simulink library "halin"  (R2021b)
settings: Solver=VariableStepAuto  StartTime=0.0  StopTime=10.0  RelTol=1e-3
undefined symbols (not defined in the file): KHAL_CAN1ABM1E2E_flg, KHAL_CAN1EPB1E2E_flg, KHAL_CAN1EPS1E2E_flg, KHAL_CAN1ESC1E2E_flg, KHAL_CAN1ESC5E2E_flg, KHAL_CAN3BMS1E2E_flg, KHAL_CAN3BMS6E2E_flg, KHAL_CAN3CCU1E2E_flg, KHAL_CAN3CCU2E2E_flg, KHAL_CAN3MCUNF1E2E_flg, KHAL_CAN3MCUNR1E2E_flg, KHAL_CAN3Shifter1E2E_flg, KHAL_CAN3Shifter2E2E_flg, KHAL_CAN6FCM2E2E_flg, KHAL_CAN6FCM4E2E_flg, TRUE
libraries: simulink x645, FVT_lib x207, hcu_lib x59
(part 19 of 23)

== system halin/HAL_IN/CAN2/IVI2/IVIPSEATHeaterCmd ==
  IVI_PSEATHeater_Cmd : Inport
  UnitConverter : DataTypeConversion  OutDataTypeStr=uint8
  VHAL_IVIPSEATHeaterCmd_enum : Outport
  wires:
  UnitConverter/1 -> VHAL_IVIPSEATHeaterCmd_enum/1
  IVI_PSEATHeater_Cmd/1 -> UnitConverter/1

== system halin/HAL_IN/CAN2/IVI2/IVIPSEATReclineCmd ==
  IVI_PSEAT_Recline_Cmd : Inport
  UnitConverter : DataTypeConversion  OutDataTypeStr=uint8
  VHAL_IVIPSEATReclineCmd_enum : Outport
  wires:
  UnitConverter/1 -> VHAL_IVIPSEATReclineCmd_enum/1
  IVI_PSEAT_Recline_Cmd/1 -> UnitConverter/1

== system halin/HAL_IN/CAN2/IVI2/IVIPSEATSlideCmd ==
  IVI_PSEAT_Slide_Cmd : Inport
  UnitConverter : DataTypeConversion  OutDataTypeStr=uint8
  VHAL_IVIPSEATSlideCmd_enum : Outport
  wires:
  UnitConverter/1 -> VHAL_IVIPSEATSlideCmd_enum/1
  IVI_PSEAT_Slide_Cmd/1 -> UnitConverter/1

== system halin/HAL_IN/CAN2/IVI2/IVIPTGModeSW ==
  IVI_PTG_Mode_SW : Inport
  UnitConverter : DataTypeConversion  OutDataTypeStr=uint8
  VHAL_IVIPTGModeSW_enum : Outport
  wires:
  UnitConverter/1 -> VHAL_IVIPTGModeSW_enum/1
  IVI_PTG_Mode_SW/1 -> UnitConverter/1

== system halin/HAL_IN/CAN2/IVI2/IVIPTGOpenHeight ==
  IVI_PTG_Open_Height : Inport
  UnitConverter : DataTypeConversion  OutDataTypeStr=uint8
  VHAL_IVIPTGOpenHeight_enum : Outport
  wires:
  UnitConverter/1 -> VHAL_IVIPTGOpenHeight_enum/1
  IVI_PTG_Open_Height/1 -> UnitConverter/1

== system halin/HAL_IN/CAN2/IVI2/IVIPTGStaSW ==
  IVI_PTG_Sta_SW : Inport
  UnitConverter : DataTypeConversion  OutDataTypeStr=uint8
  VHAL_IVIPTGStaSW_enum : Outport
  wires:
  UnitConverter/1 -> VHAL_IVIPTGStaSW_enum/1
  IVI_PTG_Sta_SW/1 -> UnitConverter/1

== system halin/HAL_IN/CAN2/IVI2/IVIPTGUSStaSW ==
  IVI_PTG_USSta_SW : Inport
  UnitConverter : DataTypeConversion  OutDataTypeStr=uint8
  VHAL_IVIPTGUSStaSW_flg : Outport
  wires:
  UnitConverter/1 -> VHAL_IVIPTGUSStaSW_flg/1
  IVI_PTG_USSta_SW/1 -> UnitConverter/1

== system halin/HAL_IN/CAN2/IVI2/IVIPWModeReq ==
  IVI_PW_Mode_Req : Inport
  UnitConverter : DataTypeConversion  OutDataTypeStr=uint8
  VHAL_IVIPWModeReq_enum : Outport
  wires:
  UnitConverter/1 -> VHAL_IVIPWModeReq_enum/1
  IVI_PW_Mode_Req/1 -> UnitConverter/1

== system halin/HAL_IN/CAN2/IVI2/IVIPwrLockSW ==
  IVI_PwrLockSW : Inport
  UnitConverter : DataTypeConversion  OutDataTypeStr=uint8
  VHAL_IVIPwrLockSW_enum : Outport
  wires:
  UnitConverter/1 -> VHAL_IVIPwrLockSW_enum/1
  IVI_PwrLockSW/1 -> UnitConverter/1

== system halin/HAL_IN/CAN2/IVI2/IVIPwroffreq ==
  IVI_Pwroff_req : Inport
  UnitConverter : DataTypeConversion  OutDataTypeStr=uint8
  VHAL_IVIPwroffreq_flg : Outport
  wires:
  UnitConverter/1 -> VHAL_IVIPwroffreq_flg/1
  IVI_Pwroff_req/1 -> UnitConverter/1

== system halin/HAL_IN/CAN2/IVI2/IVIRRDefReq ==
  IVI_RR_Def_Req : Inport
  UnitConverter : DataTypeConversion  OutDataTypeStr=uint8
  VHAL_IVIRRDefReq_flg : Outport
  wires:
  UnitConverter/1 -> VHAL_IVIRRDefReq_flg/1
  IVI_RR_Def_Req/1 -> UnitConverter/1

== system halin/HAL_IN/CAN2/IVI2/IVIReqV2L ==
  IVI_Req_V2L : Inport
  UnitConverter : DataTypeConversion  OutDataTypeStr=uint8
  VHAL_IVIReqV2L_enum : Outport
  wires:
  UnitConverter/1 -> VHAL_IVIReqV2L_enum/1
  IVI_Req_V2L/1 -> UnitConverter/1

== system halin/HAL_IN/CAN2/IVI2/IVISWCRUndefinedSta ==
  IVI_SWC_RUndefined_Sta : Inport
  UnitConverter : DataTypeConversion  OutDataTypeStr=uint8
  VHAL_IVISWCRUndefinedSta_enum : Outport
  wires:
  UnitConverter/1 -> VHAL_IVISWCRUndefinedSta_enum/1
  IVI_SWC_RUndefined_Sta/1 -> UnitConverter/1

== system halin/HAL_IN/CAN2/IVI2/IVIScreen ==
  IVI_Screen : Inport
  UnitConverter : DataTypeConversion  OutDataTypeStr=uint8
  VHAL_IVIScreen_enum : Outport
  wires:
  UnitConverter/1 -> VHAL_IVIScreen_enum/1
  IVI_Screen/1 -> UnitConverter/1

== system halin/HAL_IN/CAN2/IVI2/IVIStartChgreq ==
  IVI_Start_Chg_req : Inport
  UnitConverter : DataTypeConversion  OutDataTypeStr=uint8
  VHAL_IVIStartChgreq_flg : Outport
  wires:
  UnitConverter/1 -> VHAL_IVIStartChgreq_flg/1
  IVI_Start_Chg_req/1 -> UnitConverter/1

== system halin/HAL_IN/CAN2/IVI2/IVIStatus ==
  IVI_Status : Inport
  UnitConverter : DataTypeConversion  OutDataTypeStr=uint8
  VHAL_IVIStatus_flg : Outport
  wires:
  UnitConverter/1 -> VHAL_IVIStatus_flg/1
  IVI_Status/1 -> UnitConverter/1

== system halin/HAL_IN/CAN2/IVI2/IVIStopChgreq ==
  IVI_Stop_Chg_req : Inport
  UnitConverter : DataTypeConversion  OutDataTypeStr=uint8
  VHAL_IVIStopChgreq_flg : Outport
  wires:
  UnitConverter/1 -> VHAL_IVIStopChgreq_flg/1
  IVI_Stop_Chg_req/1 -> UnitConverter/1

== system halin/HAL_IN/CAN2/IVI2/IVITrailerCheckReqSta ==
  IVI_TrailerCheckReq_Sta : Inport
  UnitConverter : DataTypeConversion  OutDataTypeStr=uint8
  VHAL_IVITrailerCheckReqSta_flg : Outport
  wires:
  UnitConverter/1 -> VHAL_IVITrailerCheckReqSta_flg/1
  IVI_TrailerCheckReq_Sta/1 -> UnitConverter/1

== system halin/HAL_IN/CAN2/IVI2/IVITrailerModeSWSta ==
  IVI_TrailerModeSW_Sta : Inport
  UnitConverter : DataTypeConversion  OutDataTypeStr=uint8
  VHAL_IVITrailerModeSWSta_flg : Outport
  wires:
  UnitConverter/1 -> VHAL_IVITrailerModeSWSta_flg/1
  IVI_TrailerModeSW_Sta/1 -> UnitConverter/1

== system halin/HAL_IN/CAN2/IVI2/IVITriggerreq ==
  IVI_Trigger_req : Inport
  UnitConverter : DataTypeConversion  OutDataTypeStr=uint8
  VHAL_IVITriggerreq_flg : Outport
  wires:
  UnitConverter/1 -> VHAL_IVITriggerreq_flg/1
  IVI_Trigger_req/1 -> UnitConverter/1

== system halin/HAL_IN/CAN2/IVI2/IVIUnlockChgreq ==
  IVI_Unlock_Chg_req : Inport
  UnitConverter : DataTypeConversion  OutDataTypeStr=uint8
  VHAL_IVIUnlockChgreq_flg : Outport
  wires:
  UnitConverter/1 -> VHAL_IVIUnlockChgreq_flg/1
  IVI_Unlock_Chg_req/1 -> UnitConverter/1

== system halin/HAL_IN/CAN2/IVI2/IVIWIMAINSW ==
  IVI_WI_MAIN_SW : Inport
  UnitConverter : DataTypeConversion  OutDataTypeStr=uint8
  VHAL_IVIWIMAINSW_flg : Outport
  wires:
  UnitConverter/1 -> VHAL_IVIWIMAINSW_flg/1
  IVI_WI_MAIN_SW/1 -> UnitConverter/1

== system halin/HAL_IN/CAN2/IVI2/LDrvControlCommand ==
  L_Drv_ControlCommand : Inport
  UnitConverter : DataTypeConversion  OutDataTypeStr=uint8
  VHAL_LDrvControlCommand_pct : Outport
  wires:
  UnitConverter/1 -> VHAL_LDrvControlCommand_pct/1
  L_Drv_ControlCommand/1 -> UnitConverter/1

== system halin/HAL_IN/CAN2/IVI2/LPasControlCommand ==
  L_Pas_ControlCommand : Inport
  UnitConverter : DataTypeConversion  OutDataTypeStr=uint8
  VHAL_LPasControlCommand_pct : Outport
  wires:
  UnitConverter/1 -> VHAL_LPasControlCommand_pct/1
  L_Pas_ControlCommand/1 -> UnitConverter/1

== system halin/HAL_IN/CAN2/IVI2/LRLDControlCommand ==
  L_RLD_ControlCommand : Inport
  UnitConverter : DataTypeConversion  OutDataTypeStr=uint8
  VHAL_LRLDControlCommand_pct : Outport
  wires:
  UnitConverter/1 -> VHAL_LRLDControlCommand_pct/1
  L_RLD_ControlCommand/1 -> UnitConverter/1

== system halin/HAL_IN/CAN2/IVI2/LRRDControlCommand ==
  L_RRD_ControlCommand : Inport
  UnitConverter : DataTypeConversion  OutDataTypeStr=uint8
  VHAL_LRRDControlCommand_pct : Outport
  wires:
  UnitConverter/1 -> VHAL_LRRDControlCommand_pct/1
  L_RRD_ControlCommand/1 -> UnitConverter/1

== system halin/HAL_IN/CAN2/IVI2/LightShowStartReq ==
  Light_ShowStart_Req : Inport
  UnitConverter : DataTypeConversion  OutDataTypeStr=uint8
  VHAL_LightShowStartReq_flg : Outport
  wires:
  UnitConverter/1 -> VHAL_LightShowStartReq_flg/1
  Light_ShowStart_Req/1 -> UnitConverter/1

== system halin/HAL_IN/CAN2/IVI2/LightShowStopReq ==
  Light_ShowStop_Req : Inport
  UnitConverter : DataTypeConversion  OutDataTypeStr=uint8
  VHAL_LightShowStopReq_flg : Outport
  wires:
  UnitConverter/1 -> VHAL_LightShowStopReq_flg/1
  Light_ShowStop_Req/1 -> UnitConverter/1

== system halin/HAL_IN/CAN2/IVI2/MFRDNBrightReq ==
  MFRD_N_Bright_Req : Inport
  UnitConverter : DataTypeConversion  OutDataTypeStr=uint8
  VHAL_MFRDNBrightReq_pct : Outport
  wires:
  UnitConverter/1 -> VHAL_MFRDNBrightReq_pct/1
  MFRD_N_Bright_Req/1 -> UnitConverter/1

== system halin/HAL_IN/CAN2/IVI2/OFFACMODE ==
  OFF_AC_MODE : Inport
  UnitConverter : DataTypeConversion  OutDataTypeStr=uint8
  VHAL_OFFACMODE_enum : Outport
  wires:
  UnitConverter/1 -> VHAL_OFFACMODE_enum/1
  OFF_AC_MODE/1 -> UnitConverter/1

== system halin/HAL_IN/CAN2/IVI2/PSEATventreq ==
  PSEAT_vent_req : Inport
  UnitConverter : DataTypeConversion  OutDataTypeStr=uint8
  VHAL_PSEATventreq_enum : Outport
  wires:
  UnitConverter/1 -> VHAL_PSEATventreq_enum/1
  PSEAT_vent_req/1 -> UnitConverter/1

== system halin/HAL_IN/CAN2/IVI2/PerdV2L ==
  Perd_V2L : Inport
  UnitConverter : DataTypeConversion  OutDataTypeStr=uint8
  VHAL_PerdV2L_enum : Outport
  wires:
  UnitConverter/1 -> VHAL_PerdV2L_enum/1
  Perd_V2L/1 -> UnitConverter/1

== system halin/HAL_IN/CAN2/IVI2/RFogLampSW ==
  RFogLampSW : Inport
  UnitConverter : DataTypeConversion  OutDataTypeStr=uint8
  VHAL_RFogLampSW_flg : Outport
  wires:
  UnitConverter/1 -> VHAL_RFogLampSW_flg/1
  RFogLampSW/1 -> UnitConverter/1

== system halin/HAL_IN/CAN2/IVI2/RollModeSWCmd ==
  Roll_Mode_SW_Cmd : Inport
  UnitConverter : DataTypeConversion  OutDataTypeStr=uint8
  VHAL_RollModeSWCmd_enum : Outport
  wires:
  UnitConverter/1 -> VHAL_RollModeSWCmd_enum/1
  Roll_Mode_SW_Cmd/1 -> UnitConverter/1

== system halin/HAL_IN/CAN2/IVI2/RoomLampMode ==
  RoomLampMode : Inport
  UnitConverter : DataTypeConversion  OutDataTypeStr=uint8
  VHAL_RoomLampMode_flg : Outport
  wires:
  UnitConverter/1 -> VHAL_RoomLampMode_flg/1
  RoomLampMode/1 -> UnitConverter/1

== system halin/HAL_IN/CAN2/IVI2/SOCADJBUTT ==
  SOC_ADJ_BUTT : Inport
  UnitConverter : DataTypeConversion  OutDataTypeStr=uint8
  VHAL_SOCADJBUTT_flg : Outport
  wires:
  UnitConverter/1 -> VHAL_SOCADJBUTT_flg/1
  SOC_ADJ_BUTT/1 -> UnitConverter/1

== system halin/HAL_IN/CAN2/IVI2/SOCLimitSet ==
  SOC_Limit_Set : Inport
  UnitConverter : DataTypeConversion  OutDataTypeStr=uint8
  convert_in : FVT_lib/hal/convert_in  gain=2  offset=50
  VHAL_SOCLimitSet_pct : Outport
  wires:
  convert_in/1 -> VHAL_SOCLimitSet_pct/1
  UnitConverter/1 -> convert_in/1
  SOC_Limit_Set/1 -> UnitConverter/1

== system halin/HAL_IN/CAN2/IVI2/SOCV2LLimit ==
  SOC_V2LLimit : Inport
  UnitConverter : DataTypeConversion  OutDataTypeStr=uint8
  VHAL_SOCV2LLimit_pct : Outport
  wires:
  UnitConverter/1 -> VHAL_SOCV2LLimit_pct/1
  SOC_V2LLimit/1 -> UnitConverter/1

== system halin/HAL_IN/CAN2/IVI2/SchedChgStart ==
  Sched_Chg_Start : Inport
  UnitConverter : DataTypeConversion  OutDataTypeStr=uint8
  VHAL_SchedChgStart_flg : Outport
  wires:
  UnitConverter/1 -> VHAL_SchedChgStart_flg/1
  Sched_Chg_Start/1 -> UnitConverter/1

== system halin/HAL_IN/CAN2/IVI2/SchedChgStop ==
  Sched_Chg_Stop : Inport
  UnitConverter : DataTypeConversion  OutDataTypeStr=uint8
  VHAL_SchedChgStop_flg : Outport
  wires:
  UnitConverter/1 -> VHAL_SchedChgStop_flg/1
  Sched_Chg_Stop/1 -> UnitConverter/1

== system halin/HAL_IN/CAN2/IVI2/SchedChgbutt ==
  Sched_Chg_butt : Inport
  UnitConverter : DataTypeConversion  OutDataTypeStr=uint8
  VHAL_SchedChgbutt_flg : Outport
  wires:
  UnitConverter/1 -> VHAL_SchedChgbutt_flg/1
  Sched_Chg_butt/1 -> UnitConverter/1

== system halin/HAL_IN/CAN2/IVI2/SchedChglimit ==
  Sched_Chg_limit : Inport
  UnitConverter : DataTypeConversion  OutDataTypeStr=uint8
  convert_in : FVT_lib/hal/convert_in  gain=2  offset=50
  VHAL_SchedChglimit_pct : Outport
  wires:
  convert_in/1 -> VHAL_SchedChglimit_pct/1
  UnitConverter/1 -> convert_in/1
  Sched_Chg_limit/1 -> UnitConverter/1

== system halin/HAL_IN/CAN2/IVI2/SchedChgwake ==
  Sched_Chg_wake : Inport
  UnitConverter : DataTypeConversion  OutDataTypeStr=uint8
  VHAL_SchedChgwake_flg : Outport
  wires:
  UnitConverter/1 -> VHAL_SchedChgwake_flg/1
  Sched_Chg_wake/1 -> UnitConverter/1

== system halin/HAL_IN/CAN2/IVI2/SenstivityPosition ==
  SenstivityPosition : Inport
  UnitConverter : DataTypeConversion  OutDataTypeStr=uint8
  VHAL_SenstivityPosition_enum : Outport
  wires:
  UnitConverter/1 -> VHAL_SenstivityPosition_enum/1
  SenstivityPosition/1 -> UnitConverter/1

== system halin/HAL_IN/CAN2/IVI2/SetUnlockSingle ==
  SetUnlockSingle : Inport
  UnitConverter : DataTypeConversion  OutDataTypeStr=uint8
  VHAL_SetUnlockSingle_flg : Outport
  wires:
  UnitConverter/1 -> VHAL_SetUnlockSingle_flg/1
  SetUnlockSingle/1 -> UnitConverter/1

== system halin/HAL_IN/CAN2/IVI2/TCSSWCmd ==
  TCS_SW_Cmd : Inport
  UnitConverter : DataTypeConversion  OutDataTypeStr=uint8
  VHAL_TCSSWCmd_enum : Outport
  wires:
  UnitConverter/1 -> VHAL_TCSSWCmd_enum/1
  TCS_SW_Cmd/1 -> UnitConverter/1

== system halin/HAL_IN/CAN2/IVI2/TPMSCaliButt ==
  TPMS_Cali_Butt : Inport
  UnitConverter : DataTypeConversion  OutDataTypeStr=uint8
  VHAL_TPMSCaliButt_flg : Outport
  wires:
  UnitConverter/1 -> VHAL_TPMSCaliButt_flg/1
  TPMS_Cali_Butt/1 -> UnitConverter/1

== system halin/HAL_IN/CAN2/IVI2/TPMSResButt ==
  TPMS_Res_Butt : Inport
  UnitConverter : DataTypeConversion  OutDataTypeStr=uint8
  VHAL_TPMSResButt_flg : Outport
  wires:
  UnitConverter/1 -> VHAL_TPMSResButt_flg/1
  TPMS_Res_Butt/1 -> UnitConverter/1

== system halin/HAL_IN/CAN2/IVI2/TurnSwTimeSet ==
  TurnSwTimeSet : Inport
  UnitConverter : DataTypeConversion  OutDataTypeStr=uint8
  VHAL_TurnSwTimeSet_enum : Outport
  wires:
  UnitConverter/1 -> VHAL_TurnSwTimeSet_enum/1
  TurnSwTimeSet/1 -> UnitConverter/1

== system halin/HAL_IN/CAN2/IVI2/WalkawayLockSW ==
  Walkaway_Lock_SW : Inport
  UnitConverter : DataTypeConversion  OutDataTypeStr=uint8
  VHAL_WalkawayLockSW_flg : Outport
  wires:
  UnitConverter/1 -> VHAL_WalkawayLockSW_flg/1
  Walkaway_Lock_SW/1 -> UnitConverter/1

== system halin/HAL_IN/CAN2/IVI2/WlcmLightMode ==
  WlcmLight_Mode : Inport
  UnitConverter : DataTypeConversion  OutDataTypeStr=uint8
  VHAL_WlcmLightMode_enum : Outport
  wires:
  UnitConverter/1 -> VHAL_WlcmLightMode_enum/1
  WlcmLight_Mode/1 -> UnitConverter/1

== system halin/HAL_IN/CAN2/IVI2/sigAirIntenZon1Req ==
  sigAirIntenZon1Req : Inport
  UnitConverter : DataTypeConversion  OutDataTypeStr=uint8
  VHAL_sigAirIntenZon1Req_enum : Outport
  wires:
  UnitConverter/1 -> VHAL_sigAirIntenZon1Req_enum/1
  sigAirIntenZon1Req/1 -> UnitConverter/1

== system halin/HAL_IN/CAN2/IVI2/sigDfrstReq ==
  sigDfrstReq : Inport
  UnitConverter : DataTypeConversion  OutDataTypeStr=uint8
  VHAL_sigDfrstReq_flg : Outport
  wires:
  UnitConverter/1 -> VHAL_sigDfrstReq_flg/1
  sigDfrstReq/1 -> UnitConverter/1

== system halin/HAL_IN/CAN2/IVI2/sigFaceReq ==
  sigFaceReq : Inport
  UnitConverter : DataTypeConversion  OutDataTypeStr=uint8
  VHAL_sigFaceReq_flg : Outport
  wires:
  UnitConverter/1 -> VHAL_sigFaceReq_flg/1
  sigFaceReq/1 -> UnitConverter/1

== system halin/HAL_IN/CAN2/IVI2/sigFootReq ==
  sigFootReq : Inport
  UnitConverter : DataTypeConversion  OutDataTypeStr=uint8
  VHAL_sigFootReq_flg : Outport
  wires:
  UnitConverter/1 -> VHAL_sigFootReq_flg/1
  sigFootReq/1 -> UnitConverter/1

== system halin/HAL_IN/CAN2/IVI2/sigRecircReq ==
  sigRecircReq : Inport
  UnitConverter : DataTypeConversion  OutDataTypeStr=uint8
  VHAL_sigRecircReq_flg : Outport
  wires:
  UnitConverter/1 -> VHAL_sigRecircReq_flg/1
  sigRecircReq/1 -> UnitConverter/1

== system halin/HAL_IN/CAN2/IVI2/sigSetTempZon1Req ==
  sigSetTempZon1Req : Inport
  UnitConverter : DataTypeConversion  OutDataTypeStr=uint8
  convert_in : FVT_lib/hal/convert_in  gain=0.5  offset=17
  VHAL_sigSetTempZon1Req_C : Outport
  wires:
  convert_in/1 -> VHAL_sigSetTempZon1Req_C/1
  UnitConverter/1 -> convert_in/1
  sigSetTempZon1Req/1 -> UnitConverter/1

== system halin/HAL_IN/CAN2/IVI2/sigSetTempZon2Req ==
  sigSetTempZon2Req : Inport
  UnitConverter : DataTypeConversion  OutDataTypeStr=uint8
  convert_in : FVT_lib/hal/convert_in  gain=0.5  offset=17
  VHAL_sigSetTempZon2Req_C : Outport
  wires:
  convert_in/1 -> VHAL_sigSetTempZon2Req_C/1
  UnitConverter/1 -> convert_in/1
  sigSetTempZon2Req/1 -> UnitConverter/1

== system halin/HAL_IN/CAN2/IVI3/IVICLBlowerYSta ==
  IVI_CLBlower_Y_Sta : Inport
  UnitConverter : DataTypeConversion  OutDataTypeStr=uint8
  VHAL_IVICLBlowerYSta_pct : Outport
  wires:
  UnitConverter/1 -> VHAL_IVICLBlowerYSta_pct/1
  IVI_CLBlower_Y_Sta/1 -> UnitConverter/1

== system halin/HAL_IN/CAN2/IVI3/IVICLBlowerZSta ==
  IVI_CLBlower_Z_Sta : Inport
  UnitConverter : DataTypeConversion  OutDataTypeStr=uint8
  VHAL_IVICLBlowerZSta_pct : Outport
  wires:
  UnitConverter/1 -> VHAL_IVICLBlowerZSta_pct/1
  IVI_CLBlower_Z_Sta/1 -> UnitConverter/1

== system halin/HAL_IN/CAN2/IVI3/IVICRBlowerYSta ==
  IVI_CRBlower_Y_Sta : Inport
  UnitConverter : DataTypeConversion  OutDataTypeStr=uint8
  VHAL_IVICRBlowerYSta_pct : Outport
  wires:
  UnitConverter/1 -> VHAL_IVICRBlowerYSta_pct/1
  IVI_CRBlower_Y_Sta/1 -> UnitConverter/1

== system halin/HAL_IN/CAN2/IVI3/IVICRBlowerZSta ==
  IVI_CRBlower_Z_Sta : Inport
  UnitConverter : DataTypeConversion  OutDataTypeStr=uint8
  VHAL_IVICRBlowerZSta_pct : Outport
  wires:
  UnitConverter/1 -> VHAL_IVICRBlowerZSta_pct/1
  IVI_CRBlower_Z_Sta/1 -> UnitConverter/1

== system halin/HAL_IN/CAN2/IVI3/IVIDrBlowerModeSta ==
  IVI_DrBlower_Mode_Sta : Inport
  UnitConverter : DataTypeConversion  OutDataTypeStr=uint8
  VHAL_IVIDrBlowerModeSta_enum : Outport
  wires:
  UnitConverter/1 -> VHAL_IVIDrBlowerModeSta_enum/1
  IVI_DrBlower_Mode_Sta/1 -> UnitConverter/1

== system halin/HAL_IN/CAN2/IVI3/IVIDrBlowerYSta ==
  IVI_DrBlower_Y_Sta : Inport
  UnitConverter : DataTypeConversion  OutDataTypeStr=uint8
  VHAL_IVIDrBlowerYSta_pct : Outport
  wires:
  UnitConverter/1 -> VHAL_IVIDrBlowerYSta_pct/1
  IVI_DrBlower_Y_Sta/1 -> UnitConverter/1

== system halin/HAL_IN/CAN2/IVI3/IVIDrBlowerZSta ==
  IVI_DrBlower_Z_Sta : Inport
  UnitConverter : DataTypeConversion  OutDataTypeStr=uint8
  VHAL_IVIDrBlowerZSta_pct : Outport
  wires:
  UnitConverter/1 -> VHAL_IVIDrBlowerZSta_pct/1
  IVI_DrBlower_Z_Sta/1 -> UnitConverter/1

== system halin/HAL_IN/CAN2/IVI3/IVIHMICustmiFunSta ==
  IVI_HMI_CustmiFun_Sta : Inport
  UnitConverter : DataTypeConversion  OutDataTypeStr=uint8
  VHAL_IVIHMICustmiFunSta_enum : Outport
  wires:
  UnitConverter/1 -> VHAL_IVIHMICustmiFunSta_enum/1
  IVI_HMI_CustmiFun_Sta/1 -> UnitConverter/1

== system halin/HAL_IN/CAN2/IVI3/IVIHMICustmiKEYSta ==
  IVI_HMI_CustmiKEY_Sta : Inport
  UnitConverter : DataTypeConversion  OutDataTypeStr=uint8
  VHAL_IVIHMICustmiKEYSta_enum : Outport
  wires:
  UnitConverter/1 -> VHAL_IVIHMICustmiKEYSta_enum/1
  IVI_HMI_CustmiKEY_Sta/1 -> UnitConverter/1

== system halin/HAL_IN/CAN2/IVI3/IVILSEATventCmd ==
  IVI_LSEATvent_Cmd : Inport
  UnitConverter : DataTypeConversion  OutDataTypeStr=uint8
  VHAL_IVILSEATventCmd_enum : Outport
  wires:
  UnitConverter/1 -> VHAL_IVILSEATventCmd_enum/1
  IVI_LSEATvent_Cmd/1 -> UnitConverter/1

== system halin/HAL_IN/CAN2/IVI3/IVIMLFMostCmd ==
  IVI_MLFMost_Cmd : Inport
  UnitConverter : DataTypeConversion  OutDataTypeStr=uint8
  VHAL_IVIMLFMostCmd_flg : Outport
  wires:
  UnitConverter/1 -> VHAL_IVIMLFMostCmd_flg/1
  IVI_MLFMost_Cmd/1 -> UnitConverter/1

== system halin/HAL_IN/CAN2/IVI3/IVIMLFootLiftCmd ==
  IVI_MLFootLift_Cmd : Inport
  UnitConverter : DataTypeConversion  OutDataTypeStr=uint8
  VHAL_IVIMLFootLiftCmd_enum : Outport
  wires:
  UnitConverter/1 -> VHAL_IVIMLFootLiftCmd_enum/1
  IVI_MLFootLift_Cmd/1 -> UnitConverter/1

== system halin/HAL_IN/CAN2/IVI3/IVIMLNapModeCmd ==
  IVI_MLNapMode_Cmd : Inport
  UnitConverter : DataTypeConversion  OutDataTypeStr=uint8
  VHAL_IVIMLNapModeCmd_flg : Outport
  wires:
  UnitConverter/1 -> VHAL_IVIMLNapModeCmd_flg/1
  IVI_MLNapMode_Cmd/1 -> UnitConverter/1

== system halin/HAL_IN/CAN2/IVI3/IVIMLReclinerCmd ==
  IVI_MLRecliner_Cmd : Inport
  UnitConverter : DataTypeConversion  OutDataTypeStr=uint8
  VHAL_IVIMLReclinerCmd_enum : Outport
  wires:
  UnitConverter/1 -> VHAL_IVIMLReclinerCmd_enum/1
  IVI_MLRecliner_Cmd/1 -> UnitConverter/1

== system halin/HAL_IN/CAN2/IVI3/IVIMLRestoreCmd ==
  IVI_MLRestore_Cmd : Inport
  UnitConverter : DataTypeConversion  OutDataTypeStr=uint8
  VHAL_IVIMLRestoreCmd_flg : Outport
  wires:
  UnitConverter/1 -> VHAL_IVIMLRestoreCmd_flg/1
  IVI_MLRestore_Cmd/1 -> UnitConverter/1

== system halin/HAL_IN/CAN2/IVI3/IVIMLSEATventCmd ==
  IVI_MLSEATvent_Cmd : Inport
  UnitConverter : DataTypeConversion  OutDataTypeStr=uint8
  VHAL_IVIMLSEATventCmd_enum : Outport
  wires:
  UnitConverter/1 -> VHAL_IVIMLSEATventCmd_enum/1
  IVI_MLSEATvent_Cmd/1 -> UnitConverter/1

== system halin/HAL_IN/CAN2/IVI3/IVIMLSeatLiftCmd ==
  IVI_MLSeatLift_Cmd : Inport
  UnitConverter : DataTypeConversion  OutDataTypeStr=uint8
  VHAL_IVIMLSeatLiftCmd_enum : Outport
  wires:
  UnitConverter/1 -> VHAL_IVIMLSeatLiftCmd_enum/1
  IVI_MLSeatLift_Cmd/1 -> UnitConverter/1

== system halin/HAL_IN/CAN2/IVI3/IVIMLSldRestoreCmd ==
  IVI_MLSldRestore_Cmd : Inport
  UnitConverter : DataTypeConversion  OutDataTypeStr=uint8
  VHAL_IVIMLSldRestoreCmd_flg : Outport
  wires:
  UnitConverter/1 -> VHAL_IVIMLSldRestoreCmd_flg/1
  IVI_MLSldRestore_Cmd/1 -> UnitConverter/1

== system halin/HAL_IN/CAN2/IVI3/IVIMLSliderCmd ==
  IVI_MLSlider_Cmd : Inport
  UnitConverter : DataTypeConversion  OutDataTypeStr=uint8
  VHAL_IVIMLSliderCmd_enum : Outport
  wires:
  UnitConverter/1 -> VHAL_IVIMLSliderCmd_enum/1
  IVI_MLSlider_Cmd/1 -> UnitConverter/1

== system halin/HAL_IN/CAN2/IVI3/IVIMLZeroGravityCmd ==
  IVI_MLZeroGravity_Cmd : Inport
  UnitConverter : DataTypeConversion  OutDataTypeStr=uint8
  VHAL_IVIMLZeroGravityCmd_flg : Outport
  wires:
  UnitConverter/1 -> VHAL_IVIMLZeroGravityCmd_flg/1
  IVI_MLZeroGravity_Cmd/1 -> UnitConverter/1

== system halin/HAL_IN/CAN2/IVI3/IVIMRFMostCmd ==
  IVI_MRFMost_Cmd : Inport
  UnitConverter : DataTypeConversion  OutDataTypeStr=uint8
  VHAL_IVIMRFMostCmd_flg : Outport
  wires:
  UnitConverter/1 -> VHAL_IVIMRFMostCmd_flg/1
  IVI_MRFMost_Cmd/1 -> UnitConverter/1

== system halin/HAL_IN/CAN2/IVI3/IVIMRFootLiftCmd ==
  IVI_MRFootLift_Cmd : Inport
  UnitConverter : DataTypeConversion  OutDataTypeStr=uint8
  VHAL_IVIMRFootLiftCmd_enum : Outport
  wires:
  UnitConverter/1 -> VHAL_IVIMRFootLiftCmd_enum/1
  IVI_MRFootLift_Cmd/1 -> UnitConverter/1

== system halin/HAL_IN/CAN2/IVI3/IVIMRNapModeCmd ==
  IVI_MRNapMode_Cmd : Inport
  UnitConverter : DataTypeConversion  OutDataTypeStr=uint8
  VHAL_IVIMRNapModeCmd_flg : Outport
  wires:
  UnitConverter/1 -> VHAL_IVIMRNapModeCmd_flg/1
  IVI_MRNapMode_Cmd/1 -> UnitConverter/1

== system halin/HAL_IN/CAN2/IVI3/IVIMRReclinerCmd ==
  IVI_MRRecliner_Cmd : Inport
  UnitConverter : DataTypeConversion  OutDataTypeStr=uint8
  VHAL_IVIMRReclinerCmd_enum : Outport
  wires:
  UnitConverter/1 -> VHAL_IVIMRReclinerCmd_enum/1
  IVI_MRRecliner_Cmd/1 -> UnitConverter/1

== system halin/HAL_IN/CAN2/IVI3/IVIMRRestoreCmd ==
  IVI_MRRestore_Cmd : Inport
  UnitConverter : DataTypeConversion  OutDataTypeStr=uint8
  VHAL_IVIMRRestoreCmd_flg : Outport
  wires:
  UnitConverter/1 -> VHAL_IVIMRRestoreCmd_flg/1
  IVI_MRRestore_Cmd/1 -> UnitConverter/1

== system halin/HAL_IN/CAN2/IVI3/IVIMRSEATventCmd ==
  IVI_MRSEATvent_Cmd : Inport
  UnitConverter : DataTypeConversion  OutDataTypeStr=uint8
  VHAL_IVIMRSEATventCmd_enum : Outport
  wires:
  UnitConverter/1 -> VHAL_IVIMRSEATventCmd_enum/1
  IVI_MRSEATvent_Cmd/1 -> UnitConverter/1

== system halin/HAL_IN/CAN2/IVI3/IVIMRSeatLiftCmd ==
  IVI_MRSeatLift_Cmd : Inport
  UnitConverter : DataTypeConversion  OutDataTypeStr=uint8
  VHAL_IVIMRSeatLiftCmd_enum : Outport
  wires:
  UnitConverter/1 -> VHAL_IVIMRSeatLiftCmd_enum/1
  IVI_MRSeatLift_Cmd/1 -> UnitConverter/1

== system halin/HAL_IN/CAN2/IVI3/IVIMRSldRestoreCmd ==
  IVI_MRSldRestore_Cmd : Inport
  UnitConverter : DataTypeConversion  OutDataTypeStr=uint8
  VHAL_IVIMRSldRestoreCmd_flg : Outport
  wires:
  UnitConverter/1 -> VHAL_IVIMRSldRestoreCmd_flg/1
  IVI_MRSldRestore_Cmd/1 -> UnitConverter/1

== system halin/HAL_IN/CAN2/IVI3/IVIMRSliderCmd ==
  IVI_MRSlider_Cmd : Inport
  UnitConverter : DataTypeConversion  OutDataTypeStr=uint8
  VHAL_IVIMRSliderCmd_enum : Outport
  wires:
  UnitConverter/1 -> VHAL_IVIMRSliderCmd_enum/1
  IVI_MRSlider_Cmd/1 -> UnitConverter/1

== system halin/HAL_IN/CAN2/IVI3/IVIMRZeroGravityCmd ==
  IVI_MRZeroGravity_Cmd : Inport
  UnitConverter : DataTypeConversion  OutDataTypeStr=uint8
  VHAL_IVIMRZeroGravityCmd_flg : Outport
  wires:
  UnitConverter/1 -> VHAL_IVIMRZeroGravityCmd_flg/1
  IVI_MRZeroGravity_Cmd/1 -> UnitConverter/1

== system halin/HAL_IN/CAN2/IVI3/IVIPsBlowerModeSta ==
  IVI_PsBlower_Mode_Sta : Inport
  UnitConverter : DataTypeConversion  OutDataTypeStr=uint8
  VHAL_IVIPsBlowerModeSta_enum : Outport
  wires:
  UnitConverter/1 -> VHAL_IVIPsBlowerModeSta_enum/1
  IVI_PsBlower_Mode_Sta/1 -> UnitConverter/1

== system halin/HAL_IN/CAN2/IVI3/IVIPsBlowerYSta ==
  IVI_PsBlower_Y_Sta : Inport
  UnitConverter : DataTypeConversion  OutDataTypeStr=uint8
  VHAL_IVIPsBlowerYSta_pct : Outport
  wires:
  UnitConverter/1 -> VHAL_IVIPsBlowerYSta_pct/1
  IVI_PsBlower_Y_Sta/1 -> UnitConverter/1

== system halin/HAL_IN/CAN2/IVI3/IVIPsBlowerZSta ==
  IVI_PsBlower_Z_Sta : Inport
  UnitConverter : DataTypeConversion  OutDataTypeStr=uint8
  VHAL_IVIPsBlowerZSta_pct : Outport
  wires:
  UnitConverter/1 -> VHAL_IVIPsBlowerZSta_pct/1
  IVI_PsBlower_Z_Sta/1 -> UnitConverter/1

== system halin/HAL_IN/CAN2/IVI3/IVIRSEATventCmd ==
  IVI_RSEATvent_Cmd : Inport
  UnitConverter : DataTypeConversion  OutDataTypeStr=uint8
  VHAL_IVIRSEATventCmd_enum : Outport
  wires:
  UnitConverter/1 -> VHAL_IVIRSEATventCmd_enum/1
  IVI_RSEATvent_Cmd/1 -> UnitConverter/1

== system halin/HAL_IN/CAN2/IVI3/IVISnowModeCmd ==
  IVI_SnowMode_Cmd : Inport
  UnitConverter : DataTypeConversion  OutDataTypeStr=uint8
  VHAL_IVISnowModeCmd_flg : Outport
  wires:
  UnitConverter/1 -> VHAL_IVISnowModeCmd_flg/1
  IVI_SnowMode_Cmd/1 -> UnitConverter/1

== system halin/HAL_IN/CAN2/IVI3/IVIUserTakeOverAPSSta ==
  IVI_UserTakeOver_APS_Sta : Inport
  UnitConverter : DataTypeConversion  OutDataTypeStr=uint8
  VHAL_IVIUserTakeOverAPSSta_flg : Outport
  wires:
  UnitConverter/1 -> VHAL_IVIUserTakeOverAPSSta_flg/1
  IVI_UserTakeOver_APS_Sta/1 -> UnitConverter/1

== system halin/HAL_IN/CAN2/IVI3/IVIZon1WindDirSWReqSta ==
  IVI_Zon1WindDirSWReq_Sta : Inport
  UnitConverter : DataTypeConversion  OutDataTypeStr=uint8
  VHAL_IVIZon1WindDirSWReqSta_flg : Outport
  wires:
  UnitConverter/1 -> VHAL_IVIZon1WindDirSWReqSta_flg/1
  IVI_Zon1WindDirSWReq_Sta/1 -> UnitConverter/1

== system halin/HAL_IN/CAN2/METER1/METERKPHCalcu ==
  METER_KPH_Calcu : Inport
  UnitConverter : DataTypeConversion  OutDataTypeStr=uint8
  VHAL_METERKPHCalcu_kph : Outport
  wires:
  UnitConverter/1 -> VHAL_METERKPHCalcu_kph/1
  METER_KPH_Calcu/1 -> UnitConverter/1

== system halin/HAL_IN/CAN2/METER1/ODOMETER ==
  ODOMETER : Inport
  UnitConverter : DataTypeConversion  OutDataTypeStr=uint32
  convert_in : FVT_lib/hal/convert_in  gain=0.1  offset=0
  VHAL_ODOMETER_km : Outport
  wires:
  convert_in/1 -> VHAL_ODOMETER_km/1
  UnitConverter/1 -> convert_in/1
  ODOMETER/1 -> UnitConverter/1

== system halin/HAL_IN/CAN3/BMS1/BMSChckSum1 ==
  BMSChckSum_1 : Inport
  UnitConverter : DataTypeConversion  OutDataTypeStr=uint8
  VHAL_BMSChckSum1_enum : Outport
  wires:
  UnitConverter/1 -> VHAL_BMSChckSum1_enum/1
  BMSChckSum_1/1 -> UnitConverter/1

== system halin/HAL_IN/CAN3/BMS1/BMSRolCnct1 ==
  BMSRolCnct_1 : Inport
  UnitConverter : DataTypeConversion  OutDataTypeStr=uint8
  VHAL_BMSRolCnct1_enum : Outport
  wires:
  UnitConverter/1 -> VHAL_BMSRolCnct1_enum/1
  BMSRolCnct_1/1 -> UnitConverter/1

== system halin/HAL_IN/CAN3/BMS1/HVBPwrAvailChrg ==
  HVBPwrAvailChrg : Inport
  UnitConverter : DataTypeConversion  OutDataTypeStr=uint16
  convert_in : FVT_lib/hal/convert_in  gain=0.2  offset=0
  VHAL_HVBPwrAvailChrg_kW : Outport
  wires:
  convert_in/1 -> VHAL_HVBPwrAvailChrg_kW/1
  UnitConverter/1 -> convert_in/1
  HVBPwrAvailChrg/1 -> UnitConverter/1

== system halin/HAL_IN/CAN3/BMS1/HVBPwrAvailChrg30 ==
  HVBPwrAvailChrg30 : Inport
  UnitConverter : DataTypeConversion  OutDataTypeStr=uint16
  convert_in : FVT_lib/hal/convert_in  gain=0.2  offset=0
  VHAL_HVBPwrAvailChrg30_kW : Outport
  wires:
  convert_in/1 -> VHAL_HVBPwrAvailChrg30_kW/1
  UnitConverter/1 -> convert_in/1
  HVBPwrAvailChrg30/1 -> UnitConverter/1

== system halin/HAL_IN/CAN3/BMS1/HVBPwrAvailChrg60 ==
  HVBPwrAvailChrg60 : Inport
  UnitConverter : DataTypeConversion  OutDataTypeStr=uint16
  convert_in : FVT_lib/hal/convert_in  gain=0.2  offset=0
  VHAL_HVBPwrAvailChrg60_kW : Outport
  wires:
  convert_in/1 -> VHAL_HVBPwrAvailChrg60_kW/1
  UnitConverter/1 -> convert_in/1
  HVBPwrAvailChrg60/1 -> UnitConverter/1

== system halin/HAL_IN/CAN3/BMS1/HVBPwrAvailDchrg ==
  HVBPwrAvailDchrg : Inport
  UnitConverter : DataTypeConversion  OutDataTypeStr=uint16
  convert_in : FVT_lib/hal/convert_in  gain=0.2  offset=0
  VHAL_HVBPwrAvailDchrg_kW : Outport
  wires:
  convert_in/1 -> VHAL_HVBPwrAvailDchrg_kW/1
  UnitConverter/1 -> convert_in/1
  HVBPwrAvailDchrg/1 -> UnitConverter/1

== system halin/HAL_IN/CAN3/BMS1/HVBPwrAvailDchrg30 ==
  HVBPwrAvailDchrg30 : Inport
  UnitConverter : DataTypeConversion  OutDataTypeStr=uint16
  convert_in : FVT_lib/hal/convert_in  gain=0.2  offset=0
  VHAL_HVBPwrAvailDchrg30_kW : Outport
  wires:
  convert_in/1 -> VHAL_HVBPwrAvailDchrg30_kW/1
  UnitConverter/1 -> convert_in/1
  HVBPwrAvailDchrg30/1 -> UnitConverter/1

== system halin/HAL_IN/CAN3/BMS1/HVBPwrAvailDchrg60 ==
  HVBPwrAvailDchrg60 : Inport
  UnitConverter : DataTypeConversion  OutDataTypeStr=uint16
  convert_in : FVT_lib/hal/convert_in  gain=0.2  offset=0
  VHAL_HVBPwrAvailDchrg60_kW : Outport
  wires:
  convert_in/1 -> VHAL_HVBPwrAvailDchrg60_kW/1
  UnitConverter/1 -> convert_in/1
  HVBPwrAvailDchrg60/1 -> UnitConverter/1

== system halin/HAL_IN/CAN3/BMS1/HVBattCurr ==
  HVBattCurr : Inport
  UnitConverter : DataTypeConversion  OutDataTypeStr=uint16
  convert_in : FVT_lib/hal/convert_in  gain=0.1  offset=-1000
  VHAL_HVBattCurr_A : Outport
  wires:
  convert_in/1 -> VHAL_HVBattCurr_A/1
  UnitConverter/1 -> convert_in/1
  HVBattCurr/1 -> UnitConverter/1

== system halin/HAL_IN/CAN3/BMS1/HVBattVolt ==
  HVBattVolt : Inport
  UnitConverter : DataTypeConversion  OutDataTypeStr=uint16
  convert_in : FVT_lib/hal/convert_in  gain=0.1  offset=0
  VHAL_HVBattVolt_V : Outport
  wires:
  convert_in/1 -> VHAL_HVBattVolt_V/1
  UnitConverter/1 -> convert_in/1
  HVBattVolt/1 -> UnitConverter/1

== system halin/HAL_IN/CAN3/BMS3/ACChrgCurrDis ==
  ACChrgCurrDis : Inport
  UnitConverter : DataTypeConversion  OutDataTypeStr=uint16
  convert_in : FVT_lib/hal/convert_in  gain=0.1  offset=-1000
  VHAL_ACChrgCurrDis_A : Outport
  wires:
  convert_in/1 -> VHAL_ACChrgCurrDis_A/1
  UnitConverter/1 -> convert_in/1
  ACChrgCurrDis/1 -> UnitConverter/1

== system halin/HAL_IN/CAN3/BMS3/FireDetErr ==
  FireDetErr : Inport
  UnitConverter : DataTypeConversion  OutDataTypeStr=uint8
  VHAL_FireDetErr_flg : Outport
  wires:
  UnitConverter/1 -> VHAL_FireDetErr_flg/1
  FireDetErr/1 -> UnitConverter/1

== system halin/HAL_IN/CAN3/BMS3/HVBChrgPwr ==
  HVBChrgPwr : Inport
  UnitConverter : DataTypeConversion  OutDataTypeStr=uint16
  convert_in : FVT_lib/hal/convert_in  gain=0.1  offset=0
  VHAL_HVBChrgPwr_kWh : Outport
  wires:
  convert_in/1 -> VHAL_HVBChrgPwr_kWh/1
  UnitConverter/1 -> convert_in/1
  HVBChrgPwr/1 -> UnitConverter/1

== system halin/HAL_IN/CAN3/BMS3/HVBChrgPwrTotal ==
  HVBChrgPwrTotal : Inport
  UnitConverter : DataTypeConversion  OutDataTypeStr=uint32
  VHAL_HVBChrgPwrTotal_kWh : Outport
  wires:
  UnitConverter/1 -> VHAL_HVBChrgPwrTotal_kWh/1
  HVBChrgPwrTotal/1 -> UnitConverter/1

== system halin/HAL_IN/CAN3/BMS3/HVBDrvPwr ==
  HVBDrvPwr : Inport
  UnitConverter : DataTypeConversion  OutDataTypeStr=uint16
  convert_in : FVT_lib/hal/convert_in  gain=0.1  offset=0
  VHAL_HVBDrvPwr_kWh : Outport
  wires:
  convert_in/1 -> VHAL_HVBDrvPwr_kWh/1
  UnitConverter/1 -> convert_in/1
  HVBDrvPwr/1 -> UnitConverter/1

== system halin/HAL_IN/CAN3/BMS3/HVBDrvPwrTotal ==
  HVBDrvPwrTotal : Inport
  UnitConverter : DataTypeConversion  OutDataTypeStr=uint32
  VHAL_HVBDrvPwrTotal_kWh : Outport
  wires:
  UnitConverter/1 -> VHAL_HVBDrvPwrTotal_kWh/1
  HVBDrvPwrTotal/1 -> UnitConverter/1

== system halin/HAL_IN/CAN3/BMS3/HVBFullChrgPwr ==
  HVBFullChrgPwr : Inport
  UnitConverter : DataTypeConversion  OutDataTypeStr=uint16
  convert_in : FVT_lib/hal/convert_in  gain=0.1  offset=0
  VHAL_HVBFullChrgPwr_kWh : Outport
  wires:
  convert_in/1 -> VHAL_HVBFullChrgPwr_kWh/1
  UnitConverter/1 -> convert_in/1
  HVBFullChrgPwr/1 -> UnitConverter/1

== system halin/HAL_IN/CAN3/BMS3/HVBIsoImpedenceN ==
  HVBIsoImpedenceN : Inport
  UnitConverter : DataTypeConversion  OutDataTypeStr=uint16
  convert_in : FVT_lib/hal/convert_in  gain=0.01  offset=0
  VHAL_HVBIsoImpedenceN_Megaohm : Outport
  wires:
  convert_in/1 -> VHAL_HVBIsoImpedenceN_Megaohm/1
  UnitConverter/1 -> convert_in/1
  HVBIsoImpedenceN/1 -> UnitConverter/1

== system halin/HAL_IN/CAN3/BMS3/HVBIsoImpedenceP ==
  HVBIsoImpedenceP : Inport
  UnitConverter : DataTypeConversion  OutDataTypeStr=uint16
  convert_in : FVT_lib/hal/convert_in  gain=0.01  offset=0
  VHAL_HVBIsoImpedenceP_Megaohm : Outport
  wires:
  convert_in/1 -> VHAL_HVBIsoImpedenceP_Megaohm/1
  UnitConverter/1 -> convert_in/1
  HVBIsoImpedenceP/1 -> UnitConverter/1

== system halin/HAL_IN/CAN3/BMS3/HVBSOH ==
  HVBSOH : Inport
  UnitConverter : DataTypeConversion  OutDataTypeStr=uint8
  convert_in : FVT_lib/hal/convert_in  gain=0.4  offset=0
  VHAL_HVBSOH_pct : Outport
  wires:
  convert_in/1 -> VHAL_HVBSOH_pct/1
  UnitConverter/1 -> convert_in/1
  HVBSOH/1 -> UnitConverter/1

== system halin/HAL_IN/CAN3/BMS3/HVBattErr ==
  HVBattErr : Inport
  UnitConverter : DataTypeConversion  OutDataTypeStr=uint8
  VHAL_HVBattErr_flg : Outport
  wires:
  UnitConverter/1 -> VHAL_HVBattErr_flg/1
  HVBattErr/1 -> UnitConverter/1

== system halin/HAL_IN/CAN3/BMS3/HVBattPackVolt ==
  HVBattPackVolt : Inport
  UnitConverter : DataTypeConversion  OutDataTypeStr=uint16
  convert_in : FVT_lib/hal/convert_in  gain=0.1  offset=0
  VHAL_HVBattPackVolt_V : Outport
  wires:
  convert_in/1 -> VHAL_HVBattPackVolt_V/1
  UnitConverter/1 -> convert_in/1
  HVBattPackVolt/1 -> UnitConverter/1

== system halin/HAL_IN/CAN3/BMS3/HVBattSOC ==
  HVBattSOC : Inport
  UnitConverter : DataTypeConversion  OutDataTypeStr=uint8
  convert_in : FVT_lib/hal/convert_in  gain=0.4  offset=0
  VHAL_HVBattSOC_pct : Outport
  wires:
  convert_in/1 -> VHAL_HVBattSOC_pct/1
  UnitConverter/1 -> convert_in/1
  HVBattSOC/1 -> UnitConverter/1

== system halin/HAL_IN/CAN3/BMS3/HVBattSOCDis ==
  HVBattSOCDis : Inport
  UnitConverter : DataTypeConversion  OutDataTypeStr=uint8
  convert_in : FVT_lib/hal/convert_in  gain=0.4  offset=0
  VHAL_HVBattSOCDis_pct : Outport
  wires:
  convert_in/1 -> VHAL_HVBattSOCDis_pct/1
  UnitConverter/1 -> convert_in/1
  HVBattSOCDis/1 -> UnitConverter/1

== system halin/HAL_IN/CAN3/BMS3/RemainChrgTime ==
  RemainChrgTime : Inport
  UnitConverter : DataTypeConversion  OutDataTypeStr=uint16
  VHAL_RemainChrgTime_min : Outport
  wires:
  UnitConverter/1 -> VHAL_RemainChrgTime_min/1
  RemainChrgTime/1 -> UnitConverter/1

== system halin/HAL_IN/CAN3/BMS4/CellTempAvg ==
  CellTempAvg : Inport
  UnitConverter : DataTypeConversion  OutDataTypeStr=uint8
  convert_in : FVT_lib/hal/convert_in  gain=1  offset=-40
  VHAL_CellTempAvg_C : Outport
  wires:
  convert_in/1 -> VHAL_CellTempAvg_C/1
  UnitConverter/1 -> convert_in/1
  CellTempAvg/1 -> UnitConverter/1

== system halin/HAL_IN/CAN3/BMS4/HVBCellVoltMax ==
  HVBCellVoltMax : Inport
  UnitConverter : DataTypeConversion  OutDataTypeStr=uint16
  VHAL_HVBCellVoltMax_mV : Outport
  wires:
  UnitConverter/1 -> VHAL_HVBCellVoltMax_mV/1
  HVBCellVoltMax/1 -> UnitConverter/1

== system halin/HAL_IN/CAN3/BMS4/HVBCellVoltMin ==
  HVBCellVoltMin : Inport
  UnitConverter : DataTypeConversion  OutDataTypeStr=uint16
  VHAL_HVBCellVoltMin_mV : Outport
  wires:
  UnitConverter/1 -> VHAL_HVBCellVoltMin_mV/1
  HVBCellVoltMin/1 -> UnitConverter/1

== system halin/HAL_IN/CAN3/BMS4/HVBMTempMax ==
  HVBMTempMax : Inport
  UnitConverter : DataTypeConversion  OutDataTypeStr=uint8
  convert_in : FVT_lib/hal/convert_in  gain=1  offset=-40
  VHAL_HVBMTempMax_C : Outport
  wires:
  convert_in/1 -> VHAL_HVBMTempMax_C/1
  UnitConverter/1 -> convert_in/1
  HVBMTempMax/1 -> UnitConverter/1

== system halin/HAL_IN/CAN3/BMS4/HVBMTempMin ==
  HVBMTempMin : Inport
  UnitConverter : DataTypeConversion  OutDataTypeStr=uint8
  convert_in : FVT_lib/hal/convert_in  gain=1  offset=-40
  VHAL_HVBMTempMin_C : Outport
  wires:
  convert_in/1 -> VHAL_HVBMTempMin_C/1
  UnitConverter/1 -> convert_in/1
  HVBMTempMin/1 -> UnitConverter/1

== system halin/HAL_IN/CAN3/BMS4/MaxCellTempNum ==
  MaxCellTemp_Num : Inport
  UnitConverter : DataTypeConversion  OutDataTypeStr=uint8
  VHAL_MaxCellTempNum_enum : Outport
  wires:
  UnitConverter/1 -> VHAL_MaxCellTempNum_enum/1
  MaxCellTemp_Num/1 -> UnitConverter/1

== system halin/HAL_IN/CAN3/BMS4/MaxCellVoltNum ==
  MaxCellVolt_Num : Inport
  UnitConverter : DataTypeConversion  OutDataTypeStr=uint8
  VHAL_MaxCellVoltNum_enum : Outport
  wires:
  UnitConverter/1 -> VHAL_MaxCellVoltNum_enum/1
  MaxCellVolt_Num/1 -> UnitConverter/1

== system halin/HAL_IN/CAN3/BMS4/MinCellTempNum ==
  MinCellTemp_Num : Inport
  UnitConverter : DataTypeConversion  OutDataTypeStr=uint8
  VHAL_MinCellTempNum_enum : Outport
  wires:
  UnitConverter/1 -> VHAL_MinCellTempNum_enum/1
  MinCellTemp_Num/1 -> UnitConverter/1

== system halin/HAL_IN/CAN3/BMS4/MinCellVoltNum ==
  MinCellVolt_Num : Inport
  UnitConverter : DataTypeConversion  OutDataTypeStr=uint8
  VHAL_MinCellVoltNum_enum : Outport
  wires:
  UnitConverter/1 -> VHAL_MinCellVoltNum_enum/1
  MinCellVolt_Num/1 -> UnitConverter/1

== system halin/HAL_IN/CAN3/BMS5/HVInVolt ==
  HVInVolt : Inport
  UnitConverter : DataTypeConversion  OutDataTypeStr=uint16
  convert_in : FVT_lib/hal/convert_in  gain=0.1  offset=0
  VHAL_HVInVolt_V : Outport
  wires:
  convert_in/1 -> VHAL_HVInVolt_V/1
  UnitConverter/1 -> convert_in/1
  HVInVolt/1 -> UnitConverter/1

== system halin/HAL_IN/CAN3/BMS5/LVBattDet12V ==
  LVBattDet12V : Inport
  UnitConverter : DataTypeConversion  OutDataTypeStr=uint8
  convert_in : FVT_lib/hal/convert_in  gain=0.1  offset=0
  VHAL_LVBattDet12V_V : Outport
  wires:
  convert_in/1 -> VHAL_LVBattDet12V_V/1
  UnitConverter/1 -> convert_in/1
  LVBattDet12V/1 -> UnitConverter/1

== system halin/HAL_IN/CAN3/BMS5/OBCACCSLimit ==
  OBCACCSLimit : Inport
  UnitConverter : DataTypeConversion  OutDataTypeStr=uint8
  VHAL_OBCACCSLimit_A : Outport
  wires:
  UnitConverter/1 -> VHAL_OBCACCSLimit_A/1
  OBCACCSLimit/1 -> UnitConverter/1

== system halin/HAL_IN/CAN3/BMS5/OBCDCCurLm ==
  OBCDCCurLm : Inport
  UnitConverter : DataTypeConversion  OutDataTypeStr=uint16
  convert_in : FVT_lib/hal/convert_in  gain=0.1  offset=-25.5
  VHAL_OBCDCCurLm_A : Outport
  wires:
  convert_in/1 -> VHAL_OBCDCCurLm_A/1
  UnitConverter/1 -> convert_in/1
  OBCDCCurLm/1 -> UnitConverter/1

== system halin/HAL_IN/CAN3/BMS5/OBCDCVoltLm ==
  OBCDCVoltLm : Inport
  UnitConverter : DataTypeConversion  OutDataTypeStr=uint16
  convert_in : FVT_lib/hal/convert_in  gain=0.1  offset=0
  VHAL_OBCDCVoltLm_V : Outport
  wires:
  convert_in/1 -> VHAL_OBCDCVoltLm_V/1
  UnitConverter/1 -> convert_in/1
  OBCDCVoltLm/1 -> UnitConverter/1

== system halin/HAL_IN/CAN3/BMS6/BMSChckSum ==
  BMSChckSum : Inport
  UnitConverter : DataTypeConversion  OutDataTypeStr=uint8
  VHAL_BMSChckSum_enum : Outport
  wires:
  UnitConverter/1 -> VHAL_BMSChckSum_enum/1
  BMSChckSum/1 -> UnitConverter/1

== system halin/HAL_IN/CAN3/BMS6/BMSREADY ==
  BMS_READY : Inport
  UnitConverter : DataTypeConversion  OutDataTypeStr=uint8
  VHAL_BMSREADY_flg : Outport
  wires:
  UnitConverter/1 -> VHAL_BMSREADY_flg/1
  BMS_READY/1 -> UnitConverter/1

== system halin/HAL_IN/CAN3/BMS6/BMSRolCnct ==
  BMSRolCnct : Inport
  UnitConverter : DataTypeConversion  OutDataTypeStr=uint8
  VHAL_BMSRolCnct_enum : Outport
  wires:
  UnitConverter/1 -> VHAL_BMSRolCnct_enum/1
  BMSRolCnct/1 -> UnitConverter/1

== system halin/HAL_IN/CAN3/BMS6/BMSWarn1 ==
  BMS_Warn_1 : Inport
  UnitConverter : DataTypeConversion  OutDataTypeStr=uint8
  VHAL_BMSWarn1_flg : Outport
  wires:
  UnitConverter/1 -> VHAL_BMSWarn1_flg/1
  BMS_Warn_1/1 -> UnitConverter/1

== system halin/HAL_IN/CAN3/BMS6/BMSWarn2 ==
  BMS_Warn_2 : Inport
  UnitConverter : DataTypeConversion  OutDataTypeStr=uint8
  VHAL_BMSWarn2_flg : Outport
  wires:
  UnitConverter/1 -> VHAL_BMSWarn2_flg/1
  BMS_Warn_2/1 -> UnitConverter/1

== system halin/HAL_IN/CAN3/BMS6/BMSWarn3 ==
  BMS_Warn_3 : Inport
  UnitConverter : DataTypeConversion  OutDataTypeStr=uint8
  VHAL_BMSWarn3_flg : Outport
  wires:
  UnitConverter/1 -> VHAL_BMSWarn3_flg/1
  BMS_Warn_3/1 -> UnitConverter/1

== system halin/HAL_IN/CAN3/BMS6/BMSWarn4 ==
  BMS_Warn_4 : Inport
  UnitConverter : DataTypeConversion  OutDataTypeStr=uint8
  VHAL_BMSWarn4_flg : Outport
  wires:
  UnitConverter/1 -> VHAL_BMSWarn4_flg/1
  BMS_Warn_4/1 -> UnitConverter/1

== system halin/HAL_IN/CAN3/BMS6/BMSWarn5 ==
  BMS_Warn_5 : Inport
  UnitConverter : DataTypeConversion  OutDataTypeStr=uint8
  VHAL_BMSWarn5_flg : Outport
  wires:
  UnitConverter/1 -> VHAL_BMSWarn5_flg/1
  BMS_Warn_5/1 -> UnitConverter/1

== system halin/HAL_IN/CAN3/BMS6/BMSWarn6 ==
  BMS_Warn_6 : Inport
  UnitConverter : DataTypeConversion  OutDataTypeStr=uint8
  VHAL_BMSWarn6_flg : Outport
  wires:
  UnitConverter/1 -> VHAL_BMSWarn6_flg/1
  BMS_Warn_6/1 -> UnitConverter/1

== system halin/HAL_IN/CAN3/BMS6/BMSWarn7 ==
  BMS_Warn_7 : Inport
  UnitConverter : DataTypeConversion  OutDataTypeStr=uint8
  VHAL_BMSWarn7_flg : Outport
  wires:
  UnitConverter/1 -> VHAL_BMSWarn7_flg/1
  BMS_Warn_7/1 -> UnitConverter/1

== system halin/HAL_IN/CAN3/BMS6/BMSWarn8 ==
  BMS_Warn_8 : Inport
  UnitConverter : DataTypeConversion  OutDataTypeStr=uint8
  VHAL_BMSWarn8_flg : Outport
  wires:
  UnitConverter/1 -> VHAL_BMSWarn8_flg/1
  BMS_Warn_8/1 -> UnitConverter/1

== system halin/HAL_IN/CAN3/BMS6/ChrgInLockReq ==
  ChrgInLockReq : Inport
  UnitConverter : DataTypeConversion  OutDataTypeStr=uint8
  VHAL_ChrgInLockReq_enum : Outport
  wires:
  UnitConverter/1 -> VHAL_ChrgInLockReq_enum/1
  ChrgInLockReq/1 -> UnitConverter/1

== system halin/HAL_IN/CAN3/BMS6/ChrgPlugSta ==
  ChrgPlugSta : Inport
  UnitConverter : DataTypeConversion  OutDataTypeStr=uint8
  VHAL_ChrgPlugSta_enum : Outport
  wires:
  UnitConverter/1 -> VHAL_ChrgPlugSta_enum/1
  ChrgPlugSta/1 -> UnitConverter/1

== system halin/HAL_IN/CAN3/BMS6/DisChrgPlugErr ==
  DisChrgPlugErr : Inport
  UnitConverter : DataTypeConversion  OutDataTypeStr=uint8
  VHAL_DisChrgPlugErr_enum : Outport
  wires:
  UnitConverter/1 -> VHAL_DisChrgPlugErr_enum/1
  DisChrgPlugErr/1 -> UnitConverter/1

== system halin/HAL_IN/CAN3/BMS6/ExtChrgSta ==
  ExtChrgSta : Inport
  UnitConverter : DataTypeConversion  OutDataTypeStr=uint8
  VHAL_ExtChrgSta_enum : Outport
  wires:
  UnitConverter/1 -> VHAL_ExtChrgSta_enum/1
  ExtChrgSta/1 -> UnitConverter/1

== system halin/HAL_IN/CAN3/BMS6/HVBChrgErr ==
  HVBChrgErr : Inport
  UnitConverter : DataTypeConversion  OutDataTypeStr=uint8
  VHAL_HVBChrgErr_enum : Outport
  wires:
  UnitConverter/1 -> VHAL_HVBChrgErr_enum/1
  HVBChrgErr/1 -> UnitConverter/1

== system halin/HAL_IN/CAN3/BMS6/HVBContactorSta ==
  HVBContactorSta : Inport
  UnitConverter : DataTypeConversion  OutDataTypeStr=uint8
  VHAL_HVBContactorSta_flg : Outport
  wires:
  UnitConverter/1 -> VHAL_HVBContactorSta_flg/1
  HVBContactorSta/1 -> UnitConverter/1

== system halin/HAL_IN/CAN3/BMS6/HVBHVILErr ==
  HVBHVILErr : Inport
  UnitConverter : DataTypeConversion  OutDataTypeStr=uint8
  VHAL_HVBHVILErr_flg : Outport
  wires:
  UnitConverter/1 -> VHAL_HVBHVILErr_flg/1
  HVBHVILErr/1 -> UnitConverter/1

== system halin/HAL_IN/CAN3/BMS6/HVBOvrTempErr ==
  HVBOvrTempErr : Inport
  UnitConverter : DataTypeConversion  OutDataTypeStr=uint8
  VHAL_HVBOvrTempErr_flg : Outport
  wires:
  UnitConverter/1 -> VHAL_HVBOvrTempErr_flg/1
  HVBOvrTempErr/1 -> UnitConverter/1

== system halin/HAL_IN/CAN3/BMS6/HVBOvrTempWarn ==
  HVBOvrTempWarn : Inport
  UnitConverter : DataTypeConversion  OutDataTypeStr=uint8
  VHAL_HVBOvrTempWarn_enum : Outport
  wires:
  UnitConverter/1 -> VHAL_HVBOvrTempWarn_enum/1
  HVBOvrTempWarn/1 -> UnitConverter/1

== system halin/HAL_IN/CAN3/BMS6/HVBPreheatPrecoolSta ==
  HVBPreheatPrecoolSta : Inport
  UnitConverter : DataTypeConversion  OutDataTypeStr=uint8
  VHAL_HVBPreheatPrecoolSta_enum : Outport
  wires:
  UnitConverter/1 -> VHAL_HVBPreheatPrecoolSta_enum/1
  HVBPreheatPrecoolSta/1 -> UnitConverter/1

== system halin/HAL_IN/CAN3/BMS6/HVBattReady4Pre ==
  HVBattReady4Pre : Inport
  UnitConverter : DataTypeConversion  OutDataTypeStr=uint8
  VHAL_HVBattReady4Pre_enum : Outport
  wires:
  UnitConverter/1 -> VHAL_HVBattReady4Pre_enum/1
  HVBattReady4Pre/1 -> UnitConverter/1

== system halin/HAL_IN/CAN3/BMS6/HVILSta ==
  HVILSta : Inport
  UnitConverter : DataTypeConversion  OutDataTypeStr=uint8
  VHAL_HVILSta_flg : Outport
  wires:
  UnitConverter/1 -> VHAL_HVILSta_flg/1
  HVILSta/1 -> UnitConverter/1

== system halin/HAL_IN/CAN3/BMS6/V2LSta ==
  V2LSta : Inport
  UnitConverter : DataTypeConversion  OutDataTypeStr=uint8
  VHAL_V2LSta_enum : Outport
  wires:
  UnitConverter/1 -> VHAL_V2LSta_enum/1
  V2LSta/1 -> UnitConverter/1

== system halin/HAL_IN/CAN3/BMS8/MainRlyNegSta ==
  MainRlyNegSta : Inport
  UnitConverter : DataTypeConversion  OutDataTypeStr=uint8
  VHAL_MainRlyNegSta_enum : Outport
  wires:
  UnitConverter/1 -> VHAL_MainRlyNegSta_enum/1
  MainRlyNegSta/1 -> UnitConverter/1

== system halin/HAL_IN/CAN3/BMS8/MainRlyPosSta ==
  MainRlyPosSta : Inport
  UnitConverter : DataTypeConversion  OutDataTypeStr=uint8
  VHAL_MainRlyPosSta_enum : Outport
  wires:
  UnitConverter/1 -> VHAL_MainRlyPosSta_enum/1
  MainRlyPosSta/1 -> UnitConverter/1

== system halin/HAL_IN/CAN3/CCU1/CSCCU1 ==
  CS_CCU1 : Inport
  UnitConverter : DataTypeConversion  OutDataTypeStr=uint8
  VHAL_CSCCU1_enum : Outport
  wires:
  UnitConverter/1 -> VHAL_CSCCU1_enum/1
  CS_CCU1/1 -> UnitConverter/1

== system halin/HAL_IN/CAN3/CCU1/DCDCAuxCur ==
  DCDCAuxCur : Inport
  UnitConverter : DataTypeConversion  OutDataTypeStr=uint16
  convert_in : FVT_lib/hal/convert_in  gain=0.1  offset=0
  VHAL_DCDCAuxCur_A : Outport
  wires:
  convert_in/1 -> VHAL_DCDCAuxCur_A/1
  UnitConverter/1 -> convert_in/1
  DCDCAuxCur/1 -> UnitConverter/1

== system halin/HAL_IN/CAN3/CCU1/DCDCAuxVolt ==
  DCDCAuxVolt : Inport
  UnitConverter : DataTypeConversion  OutDataTypeStr=uint16
  convert_in : FVT_lib/hal/convert_in  gain=0.047  offset=8
  VHAL_DCDCAuxVolt_V : Outport
  wires:
  convert_in/1 -> VHAL_DCDCAuxVolt_V/1
  UnitConverter/1 -> convert_in/1
  DCDCAuxVolt/1 -> UnitConverter/1

== system halin/HAL_IN/CAN3/CCU1/DCDCHVCur ==
  DCDCHVCur : Inport
  UnitConverter : DataTypeConversion  OutDataTypeStr=uint16
  convert_in : FVT_lib/hal/convert_in  gain=0.02  offset=0
  VHAL_DCDCHVCur_A : Outport
  wires:
  convert_in/1 -> VHAL_DCDCHVCur_A/1
  UnitConverter/1 -> convert_in/1
  DCDCHVCur/1 -> UnitConverter/1

== system halin/HAL_IN/CAN3/CCU1/DCDCInVoltInf ==
  DCDCInVoltInf : Inport
  UnitConverter : DataTypeConversion  OutDataTypeStr=uint16
  convert_in : FVT_lib/hal/convert_in  gain=0.25  offset=0
  VHAL_DCDCInVoltInf_V : Outport
  wires:
  convert_in/1 -> VHAL_DCDCInVoltInf_V/1
  UnitConverter/1 -> convert_in/1
  DCDCInVoltInf/1 -> UnitConverter/1

== system halin/HAL_IN/CAN3/CCU1/DCDCPreCompleted ==
  DCDCPreCompleted : Inport
  UnitConverter : DataTypeConversion  OutDataTypeStr=uint8
  VHAL_DCDCPreCompleted_enum : Outport
  wires:
  UnitConverter/1 -> VHAL_DCDCPreCompleted_enum/1
  DCDCPreCompleted/1 -> UnitConverter/1

== system halin/HAL_IN/CAN3/CCU1/OBCDCCurrInf ==
  OBCDCCurrInf : Inport
  UnitConverter : DataTypeConversion  OutDataTypeStr=uint16
  convert_in : FVT_lib/hal/convert_in  gain=0.1  offset=-25.5
  VHAL_OBCDCCurrInf_A : Outport
  wires:
  convert_in/1 -> VHAL_OBCDCCurrInf_A/1
  UnitConverter/1 -> convert_in/1
  OBCDCCurrInf/1 -> UnitConverter/1

== system halin/HAL_IN/CAN3/CCU1/OBCDCVoltInf ==
  OBCDCVoltInf : Inport
  UnitConverter : DataTypeConversion  OutDataTypeStr=uint16
  convert_in : FVT_lib/hal/convert_in  gain=0.3  offset=0
  VHAL_OBCDCVoltInf_V : Outport
  wires:
  convert_in/1 -> VHAL_OBCDCVoltInf_V/1
  UnitConverter/1 -> convert_in/1
  OBCDCVoltInf/1 -> UnitConverter/1

== system halin/HAL_IN/CAN3/CCU1/OBCPreCompleted ==
  OBCPreCompleted : Inport
  UnitConverter : DataTypeConversion  OutDataTypeStr=uint16
  VHAL_OBCPreCompleted_enum : Outport
  wires:
  UnitConverter/1 -> VHAL_OBCPreCompleted_enum/1
  OBCPreCompleted/1 -> UnitConverter/1

== system halin/HAL_IN/CAN3/CCU1/OBCWakeup4Plugin ==
  OBCWakeup4Plugin : Inport
  UnitConverter : DataTypeConversion  OutDataTypeStr=uint8
  VHAL_OBCWakeup4Plugin_flg : Outport
  wires:
  UnitConverter/1 -> VHAL_OBCWakeup4Plugin_flg/1
  OBCWakeup4Plugin/1 -> UnitConverter/1

== system halin/HAL_IN/CAN3/CCU1/RCCCU1 ==
  RC_CCU1 : Inport
  UnitConverter : DataTypeConversion  OutDataTypeStr=uint8
  VHAL_RCCCU1_enum : Outport
  wires:
  UnitConverter/1 -> VHAL_RCCCU1_enum/1
  RC_CCU1/1 -> UnitConverter/1
